simulink model "FeedbackLin"  (R2016a)
settings: Solver=ode45  StartTime=0.0  StopTime=2*Tpasso  FixedStep=1e-4  RelTol=1e-5
values from neighbouring files (symbols this model uses):
  Bm = 1e-4    (= 0.0001)    [runTests.m]
  cm = [c1; c2; c3; c4; c5]    [runTests.m]
  Cphi = 1    [runTests.m]
  cr = [c1; c2; c3; c4; c5]    [runTests.m]
  dQ0 = [dQ10; dQ20; dQ30; dQ40; dQ50]    [runNoErrorNoNoiseNoIncNoFext.m]    (also in runTests.m = zeros(5,1))
  gait = 1    [runTests.m]
  gm = g    (= 9.81)    [runTests.m]
  gr = g    (= 9.81)    [runTests.m]
  Im = [I1; I2; I3; I4; I5]    [runTests.m]
  Ir = [I1; I2; I3; I4; I5]    [runTests.m]
  Jm = 5e-3    (= 0.005)    [runTests.m]
  Kt = 0.1    [runTests.m]
  La = 1e-3    (= 0.001)    [runTests.m]
  LambdaFL = [150; 150; 150; 150]    [runTests.m]
  lm = [l1; l2; l3; l4; l5]    [runTests.m]
  lr = [l1; l2; l3; l4; l5]    [runTests.m]
  mInc = tan(Inc*pi/180)    [runTests.m]
  mm = [m1; m2; m3; m4; m5]    [runTests.m]
  mr = [m1; m2; m3; m4; m5]    [runTests.m]
  pertAmp = 0    [runTests.m]
  pertDur = 0    [runTests.m]
  pertStep = 0    [runTests.m]
  Q0 = [Q10; Q20; Q30; Q40; Q50]    [runNoErrorNoNoiseNoIncNoFext.m]    (also in runTests.m = [pi/2 - pi/10; pi/5; 2*pi-pi/10; pi+pi/10; -pi/4.5])
  Ra = 1    [runTests.m]
  Tpasso = 0.35    [runTests.m]
  TsC = 0.003    [runTests.m]
  TsPID = 1/1000    (= 0.001)    [runTests.m]
  useNoise = false    [runTests.m]
undefined symbols (not defined in the file or in its folder): curStep, Rp1, Rp2
libraries: simulink x8, commrandsrc3 x2
(part 2 of 3)

== matlab function FeedbackLin/calcU ==
  data: Ut output; dQ input; Q input; Yd input; dYd input; ddYd input; Cphi parameter; mm parameter; cm parameter; lm parameter; Im parameter; gm parameter; LambdaFL parameter; Y_bar output
function [Ut, Y_bar] = calcControl(dQ, Q, Yd, dYd, ddYd, Cphi, mm, cm, lm, Im, gm, LambdaFL)
    Mest = zeros(5,5);
    Cest = zeros(5,5);
    Gest = zeros(5,1);
    
    %Control matrices
    diffCq_q    = zeros(4, 5);
    diffLfCq_q  = zeros(4, 5);
    diffLfCq_dq = zeros(4, 5);
    
    %Matrix that appliest 0 torque to joint 1 and the corresponding torque
    %to all other joints.
    Bcontrol = [[0, 0, 0, 0]; ...
                [1, 0, 0, 0]; ...
                [0, 1, 0, 0]; ...
                [0, 0, 1, 0]; ...
                [0, 0, 0, 1]];    
    
    
    %Model Parameters 
    m1 = mm(1);
    m2 = mm(2);
    m3 = mm(3);
    m4 = mm(4);
    m5 = mm(5);

    c1 = cm(1);
    c2 = cm(2);
    c3 = cm(3);
    c4 = cm(4);
    c5 = cm(5);

    l1 = lm(1);
    l2 = lm(2);
    l3 = lm(3);
    l4 = lm(4);
    l5 = lm(5);

    g = gm;

    I1 = Im(1);
    I2 = Im(2);
    I3 = Im(3);
    I4 = Im(4);
    I5 = Im(5);
    
    %Current positions
    q1 = Q(1);
    q2 = Q(2);
    q3 = Q(3);
    q4 = Q(4);
    q5 = Q(5);
    
    dq1 = dQ(1);
    dq2 = dQ(2);
    dq3 = dQ(3);
    dq4 = dQ(4);
    dq5 = dQ(5);
    
    Mest(1, 1) = I1 + I2 + I3 + I4 + I5 + c1^2*m1 + c2^2*m2 + c3^2*m3 + c4^2*m4 + c5^2*m5 + l1^2*m1 + l1^2*m2 + l1^2*m3 + l2^2*m2 + l1^2*m4 + l2^2*m3 + l1^2*m5 + l2^2*m4 + l2^2*m5 + l4^2*m5 - 2*c1*l1*m1 - 2*c2*l2*m2 + 2*c5*l1*m5*cos(q2 + q3 + q4 + q5) + 2*c3*l1*m3*cos(q2 + q3) + 2*c4*l2*m4*cos(q3 + q4) + 2*l2*l4*m5*cos(q3 + q4) - 2*c2*l1*m2*cos(q2) + 2*c3*l2*m3*cos(q3) + 2*c5*l4*m5*cos(q5) + 2*l1*l2*m2*cos(q2) + 2*l1*l2*m3*cos(q2) + 2*l1*l2*m4*cos(q2) + 2*l1*l2*m5*cos(q2) + 2*c4*l1*m4*cos(q2 + q3 + q4) + 2*c5*l2*m5*cos(q3 + q4 + q5) + 2*l1*l4*m5*cos(q2 + q3 + q4);
    Mest(2, 1) = I2 + I3 + I4 + I5 + c2^2*m2 + c3^2*m3 + c4^2*m4 + c5^2*m5 + l2^2*m2 + l2^2*m3 + l2^2*m4 + l2^2*m5 + l4^2*m5 - 2*c2*l2*m2 + c5*l1*m5*cos(q2 + q3 + q4 + q5) + c3*l1*m3*cos(q2 + q3) + 2*c4*l2*m4*cos(q3 + q4) + 2*l2*l4*m5*cos(q3 + q4) - c2*l1*m2*cos(q2) + 2*c3*l2*m3*cos(q3) + 2*c5*l4*m5*cos(q5) + l1*l2*m2*cos(q2) + l1*l2*m3*cos(q2) + l1*l2*m4*cos(q2) + l1*l2*m5*cos(q2) + c4*l1*m4*cos(q2 + q3 + q4) + 2*c5*l2*m5*cos(q3 + q4 + q5) + l1*l4*m5*cos(q2 + q3 + q4);
    Mest(3, 1) = I3 + I4 + I5 + c3^2*m3 + c4^2*m4 + c5^2*m5 + l4^2*m5 + c5*l1*m5*cos(q2 + q3 + q4 + q5) + c3*l1*m3*cos(q2 + q3) + c4*l2*m4*cos(q3 + q4) + l2*l4*m5*cos(q3 + q4) + c3*l2*m3*cos(q3) + 2*c5*l4*m5*cos(q5) + c4*l1*m4*cos(q2 + q3 + q4) + c5*l2*m5*cos(q3 + q4 + q5) + l1*l4*m5*cos(q2 + q3 + q4);
    Mest(4, 1) = I4 + I5 + c4^2*m4 + c5^2*m5 + l4^2*m5 + c5*l1*m5*cos(q2 + q3 + q4 + q5) + c4*l2*m4*cos(q3 + q4) + l2*l4*m5*cos(q3 + q4) + 2*c5*l4*m5*cos(q5) + c4*l1*m4*cos(q2 + q3 + q4) + c5*l2*m5*cos(q3 + q4 + q5) + l1*l4*m5*cos(q2 + q3 + q4);
    Mest(5, 1) = I5 + c5^2*m5 + c5*l1*m5*cos(q2 + q3 + q4 + q5) + c5*l4*m5*cos(q5) + c5*l2*m5*cos(q3 + q4 + q5);
    Mest(1, 2) = I2 + I3 + I4 + I5 + c2^2*m2 + c3^2*m3 + c4^2*m4 + c5^2*m5 + l2^2*m2 + l2^2*m3 + l2^2*m4 + l2^2*m5 + l4^2*m5 - 2*c2*l2*m2 + c5*l1*m5*cos(q2 + q3 + q4 + q5) + c3*l1*m3*cos(q2 + q3) + 2*c4*l2*m4*cos(q3 + q4) + 2*l2*l4*m5*cos(q3 + q4) - c2*l1*m2*cos(q2) + 2*c3*l2*m3*cos(q3) + 2*c5*l4*m5*cos(q5) + l1*l2*m2*cos(q2) + l1*l2*m3*cos(q2) + l1*l2*m4*cos(q2) + l1*l2*m5*cos(q2) + c4*l1*m4*cos(q2 + q3 + q4) + 2*c5*l2*m5*cos(q3 + q4 + q5) + l1*l4*m5*cos(q2 + q3 + q4);
    Mest(2, 2) = I2 + I3 + I4 + I5 + c2^2*m2 + c3^2*m3 + c4^2*m4 + c5^2*m5 + l2^2*m2 + l2^2*m3 + l2^2*m4 + l2^2*m5 + l4^2*m5 - 2*c2*l2*m2 + 2*c4*l2*m4*cos(q3 + q4) + 2*l2*l4*m5*cos(q3 + q4) + 2*c3*l2*m3*cos(q3) + 2*c5*l4*m5*cos(q5) + 2*c5*l2*m5*cos(q3 + q4 + q5);
    Mest(3, 2) = I3 + I4 + I5 + c3^2*m3 + c4^2*m4 + c5^2*m5 + l4^2*m5 + c4*l2*m4*cos(q3 + q4) + l2*l4*m5*cos(q3 + q4) + c3*l2*m3*cos(q3) + 2*c5*l4*m5*cos(q5) + c5*l2*m5*cos(q3 + q4 + q5);
    Mest(4, 2) = I4 + I5 + c4^2*m4 + c5^2*m5 + l4^2*m5 + c4*l2*m4*cos(q3 + q4) + l2*l4*m5*cos(q3 + q4) + 2*c5*l4*m5*cos(q5) + c5*l2*m5*cos(q3 + q4 + q5);
    Mest(5, 2) = I5 + c5^2*m5 + c5*l4*m5*cos(q5) + c5*l2*m5*cos(q3 + q4 + q5);
    Mest(1, 3) = I3 + I4 + I5 + c3^2*m3 + c4^2*m4 + c5^2*m5 + l4^2*m5 + c5*l1*m5*cos(q2 + q3 + q4 + q5) + c3*l1*m3*cos(q2 + q3) + c4*l2*m4*cos(q3 + q4) + l2*l4*m5*cos(q3 + q4) + c3*l2*m3*cos(q3) + 2*c5*l4*m5*cos(q5) + c4*l1*m4*cos(q2 + q3 + q4) + c5*l2*m5*cos(q3 + q4 + q5) + l1*l4*m5*cos(q2 + q3 + q4);
    Mest(2, 3) = I3 + I4 + I5 + c3^2*m3 + c4^2*m4 + c5^2*m5 + l4^2*m5 + c4*l2*m4*cos(q3 + q4) + l2*l4*m5*cos(q3 + q4) + c3*l2*m3*cos(q3) + 2*c5*l4*m5*cos(q5) + c5*l2*m5*cos(q3 + q4 + q5);
    Mest(3, 3) = I3 + I4 + I5 + c3^2*m3 + c4^2*m4 + c5^2*m5 + l4^2*m5 + 2*c5*l4*m5*cos(q5);
    Mest(4, 3) = I4 + I5 + c4^2*m4 + c5^2*m5 + l4^2*m5 + 2*c5*l4*m5*cos(q5);
    Mest(5, 3) = I5 + c5^2*m5 + c5*l4*m5*cos(q5);
    Mest(1, 4) = I4 + I5 + c4^2*m4 + c5^2*m5 + l4^2*m5 + c5*l1*m5*cos(q2 + q3 + q4 + q5) + c4*l2*m4*cos(q3 + q4) + l2*l4*m5*cos(q3 + q4) + 2*c5*l4*m5*cos(q5) + c4*l1*m4*cos(q2 + q3 + q4) + c5*l2*m5*cos(q3 + q4 + q5) + l1*l4*m5*cos(q2 + q3 + q4);
    Mest(2, 4) = I4 + I5 + c4^2*m4 + c5^2*m5 + l4^2*m5 + c4*l2*m4*cos(q3 + q4) + l2*l4*m5*cos(q3 + q4) + 2*c5*l4*m5*cos(q5) + c5*l2*m5*cos(q3 + q4 + q5);
    Mest(3, 4) = I4 + I5 + c4^2*m4 + c5^2*m5 + l4^2*m5 + 2*c5*l4*m5*cos(q5);
    Mest(4, 4) = I4 + I5 + c4^2*m4 + c5^2*m5 + l4^2*m5 + 2*c5*l4*m5*cos(q5);
    Mest(5, 4) = I5 + c5^2*m5 + c5*l4*m5*cos(q5);
    Mest(1, 5) = I5 + c5^2*m5 + c5*l1*m5*cos(q2 + q3 + q4 + q5) + c5*l4*m5*cos(q5) + c5*l2*m5*cos(q3 + q4 + q5);
    Mest(2, 5) = I5 + c5^2*m5 + c5*l4*m5*cos(q5) + c5*l2*m5*cos(q3 + q4 + q5);
    Mest(3, 5) = I5 + c5^2*m5 + c5*l4*m5*cos(q5);
    Mest(4, 5) = I5 + c5^2*m5 + c5*l4*m5*cos(q5);
    Mest(5, 5) = I5 + c5^2*m5;
  
    Gest(1, 1) = g*(m3*(l2*cos(q1 + q2) + l1*cos(q1) + c3*cos(q1 + q2 + q3)) + m5*(l4*cos(q1 + q2 + q3 + q4) + l2*cos(q1 + q2) + l1*cos(q1) + c5*cos(q1 + q2 + q3 + q4 + q5)) - m2*(cos(q1 + q2)*(c2 - l2) - l1*cos(q1)) + m4*(c4*cos(q1 + q2 + q3 + q4) + l2*cos(q1 + q2) + l1*cos(q1)) - m1*cos(q1)*(c1 - l1));
    Gest(2, 1) = g*(m3*(l2*cos(q1 + q2) + c3*cos(q1 + q2 + q3)) + m5*(l4*cos(q1 + q2 + q3 + q4) + l2*cos(q1 + q2) + c5*cos(q1 + q2 + q3 + q4 + q5)) + m4*(c4*cos(q1 + q2 + q3 + q4) + l2*cos(q1 + q2)) - m2*cos(q1 + q2)*(c2 - l2));
    Gest(3, 1) = g*(m5*(l4*cos(q1 + q2 + q3 + q4) + c5*cos(q1 + q2 + q3 + q4 + q5)) + c3*m3*cos(q1 + q2 + q3) + c4*m4*cos(q1 + q2 + q3 + q4));
    Gest(4, 1) = g*(m5*(l4*cos(q1 + q2 + q3 + q4) + c5*cos(q1 + q2 + q3 + q4 + q5)) + c4*m4*cos(q1 + q2 + q3 + q4));
    Gest(5, 1) = c5*g*m5*cos(q1 + q2 + q3 + q4 + q5);
    
    Cest(1, 1) = c2*dq2*l1*m2*sin(q2) - c4*dq3*l1*m4*sin(q2 + q3 + q4) - c4*dq4*l1*m4*sin(q2 + q3 + q4) - c5*dq3*l2*m5*sin(q3 + q4 + q5) - c5*dq4*l2*m5*sin(q3 + q4 + q5) - c5*dq5*l2*m5*sin(q3 + q4 + q5) - dq2*l1*l4*m5*sin(q2 + q3 + q4) - dq3*l1*l4*m5*sin(q2 + q3 + q4) - dq4*l1*l4*m5*sin(q2 + q3 + q4) - c5*dq2*l1*m5*sin(q2 + q3 + q4 + q5) - c5*dq3*l1*m5*sin(q2 + q3 + q4 + q5) - c5*dq4*l1*m5*sin(q2 + q3 + q4 + q5) - c5*dq5*l1*m5*sin(q2 + q3 + q4 + q5) - c3*dq2*l1*m3*sin(q2 + q3) - c3*dq3*l1*m3*sin(q2 + q3) - c4*dq3*l2*m4*sin(q3 + q4) - c4*dq4*l2*m4*sin(q3 + q4) - dq3*l2*l4*m5*sin(q3 + q4) - dq4*l2*l4*m5*sin(q3 + q4) - c4*dq2*l1*m4*sin(q2 + q3 + q4) - c3*dq3*l2*m3*sin(q3) - c5*dq5*l4*m5*sin(q5) - dq2*l1*l2*m2*sin(q2) - dq2*l1*l2*m3*sin(q2) - dq2*l1*l2*m4*sin(q2) - dq2*l1*l2*m5*sin(q2);
    Cest(2, 1) = c4*dq1*l1*m4*sin(q2 + q3 + q4) - c5*dq3*l2*m5*sin(q3 + q4 + q5) - c5*dq4*l2*m5*sin(q3 + q4 + q5) - c5*dq5*l2*m5*sin(q3 + q4 + q5) + dq1*l1*l4*m5*sin(q2 + q3 + q4) + c5*dq1*l1*m5*sin(q2 + q3 + q4 + q5) + c3*dq1*l1*m3*sin(q2 + q3) - c4*dq3*l2*m4*sin(q3 + q4) - c4*dq4*l2*m4*sin(q3 + q4) - dq3*l2*l4*m5*sin(q3 + q4) - dq4*l2*l4*m5*sin(q3 + q4) - c2*dq1*l1*m2*sin(q2) - c3*dq3*l2*m3*sin(q3) - c5*dq5*l4*m5*sin(q5) + dq1*l1*l2*m2*sin(q2) + dq1*l1*l2*m3*sin(q2) + dq1*l1*l2*m4*sin(q2) + dq1*l1*l2*m5*sin(q2);
    Cest(3, 1) = c4*dq1*l1*m4*sin(q2 + q3 + q4) + c5*dq1*l2*m5*sin(q3 + q4 + q5) + c5*dq2*l2*m5*sin(q3 + q4 + q5) + dq1*l1*l4*m5*sin(q2 + q3 + q4) + c5*dq1*l1*m5*sin(q2 + q3 + q4 + q5) + c3*dq1*l1*m3*sin(q2 + q3) + c4*dq1*l2*m4*sin(q3 + q4) + c4*dq2*l2*m4*sin(q3 + q4) + dq1*l2*l4*m5*sin(q3 + q4) + dq2*l2*l4*m5*sin(q3 + q4) + c3*dq1*l2*m3*sin(q3) + c3*dq2*l2*m3*sin(q3) - c5*dq5*l4*m5*sin(q5);
    Cest(4, 1) = c4*dq1*l1*m4*sin(q2 + q3 + q4) + c5*dq1*l2*m5*sin(q3 + q4 + q5) + c5*dq2*l2*m5*sin(q3 + q4 + q5) + dq1*l1*l4*m5*sin(q2 + q3 + q4) + c5*dq1*l1*m5*sin(q2 + q3 + q4 + q5) + c4*dq1*l2*m4*sin(q3 + q4) + c4*dq2*l2*m4*sin(q3 + q4) + dq1*l2*l4*m5*sin(q3 + q4) + dq2*l2*l4*m5*sin(q3 + q4) - c5*dq5*l4*m5*sin(q5);
    Cest(5, 1) = c5*m5*(dq1*l4*sin(q5) + dq2*l4*sin(q5) + dq3*l4*sin(q5) + dq4*l4*sin(q5) + dq1*l2*sin(q3 + q4 + q5) + dq2*l2*sin(q3 + q4 + q5) + dq1*l1*sin(q2 + q3 + q4 + q5));
    Cest(1, 2) = c2*dq1*l1*m2*sin(q2) - c4*dq2*l1*m4*sin(q2 + q3 + q4) - c4*dq3*l1*m4*sin(q2 + q3 + q4) - c4*dq4*l1*m4*sin(q2 + q3 + q4) - c5*dq3*l2*m5*sin(q3 + q4 + q5) - c5*dq4*l2*m5*sin(q3 + q4 + q5) - c5*dq5*l2*m5*sin(q3 + q4 + q5) - dq1*l1*l4*m5*sin(q2 + q3 + q4) - dq2*l1*l4*m5*sin(q2 + q3 + q4) - dq3*l1*l4*m5*sin(q2 + q3 + q4) - dq4*l1*l4*m5*sin(q2 + q3 + q4) - c5*dq1*l1*m5*sin(q2 + q3 + q4 + q5) - c5*dq2*l1*m5*sin(q2 + q3 + q4 + q5) - c5*dq3*l1*m5*sin(q2 + q3 + q4 + q5) - c5*dq4*l1*m5*sin(q2 + q3 + q4 + q5) - c5*dq5*l1*m5*sin(q2 + q3 + q4 + q5) - c3*dq1*l1*m3*sin(q2 + q3) - c3*dq2*l1*m3*sin(q2 + q3) - c3*dq3*l1*m3*sin(q2 + q3) - c4*dq3*l2*m4*sin(q3 + q4) - c4*dq4*l2*m4*sin(q3 + q4) - dq3*l2*l4*m5*sin(q3 + q4) - dq4*l2*l4*m5*sin(q3 + q4) - c4*dq1*l1*m4*sin(q2 + q3 + q4) + c2*dq2*l1*m2*sin(q2) - c3*dq3*l2*m3*sin(q3) - c5*dq5*l4*m5*sin(q5) - dq1*l1*l2*m2*sin(q2) - dq1*l1*l2*m3*sin(q2) - dq2*l1*l2*m2*sin(q2) - dq1*l1*l2*m4*sin(q2) - dq2*l1*l2*m3*sin(q2) - dq1*l1*l2*m5*sin(q2) - dq2*l1*l2*m4*sin(q2) - dq2*l1*l2*m5*sin(q2);
    Cest(2, 2) = - dq4*l2*(c5*m5*sin(q3 + q4 + q5) + c4*m4*sin(q3 + q4) + l4*m5*sin(q3 + q4)) - dq3*l2*(c3*m3*sin(q3) + c5*m5*sin(q3 + q4 + q5) + c4*m4*sin(q3 + q4) + l4*m5*sin(q3 + q4)) - c5*dq5*m5*(l4*sin(q5) + l2*sin(q3 + q4 + q5));
    Cest(3, 2) = c5*dq1*l2*m5*sin(q3 + q4 + q5) + c5*dq2*l2*m5*sin(q3 + q4 + q5) + c4*dq1*l2*m4*sin(q3 + q4) + c4*dq2*l2*m4*sin(q3 + q4) + dq1*l2*l4*m5*sin(q3 + q4) + dq2*l2*l4*m5*sin(q3 + q4) + c3*dq1*l2*m3*sin(q3) + c3*dq2*l2*m3*sin(q3) - c5*dq5*l4*m5*sin(q5);
    Cest(4, 2) = c5*dq1*l2*m5*sin(q3 + q4 + q5) + c5*dq2*l2*m5*sin(q3 + q4 + q5) + c4*dq1*l2*m4*sin(q3 + q4) + c4*dq2*l2*m4*sin(q3 + q4) + dq1*l2*l4*m5*sin(q3 + q4) + dq2*l2*l4*m5*sin(q3 + q4) - c5*dq5*l4*m5*sin(q5);
    Cest(5, 2) = c5*m5*(dq1*l4*sin(q5) + dq2*l4*sin(q5) + dq3*l4*sin(q5) + dq4*l4*sin(q5) + dq1*l2*sin(q3 + q4 + q5) + dq2*l2*sin(q3 + q4 + q5));
    Cest(1, 3) = - c4*dq1*l1*m4*sin(q2 + q3 + q4) - c4*dq2*l1*m4*sin(q2 + q3 + q4) - c4*dq3*l1*m4*sin(q2 + q3 + q4) - c4*dq4*l1*m4*sin(q2 + q3 + q4) - c5*dq1*l2*m5*sin(q3 + q4 + q5) - c5*dq2*l2*m5*sin(q3 + q4 + q5) - c5*dq3*l2*m5*sin(q3 + q4 + q5) - c5*dq4*l2*m5*sin(q3 + q4 + q5) - c5*dq5*l2*m5*sin(q3 + q4 + q5) - dq1*l1*l4*m5*sin(q2 + q3 + q4) - dq2*l1*l4*m5*sin(q2 + q3 + q4) - dq3*l1*l4*m5*sin(q2 + q3 + q4) - dq4*l1*l4*m5*sin(q2 + q3 + q4) - c5*dq1*l1*m5*sin(q2 + q3 + q4 + q5) - c5*dq2*l1*m5*sin(q2 + q3 + q4 + q5) - c5*dq3*l1*m5*sin(q2 + q3 + q4 + q5) - c5*dq4*l1*m5*sin(q2 + q3 + q4 + q5) - c5*dq5*l1*m5*sin(q2 + q3 + q4 + q5) - c3*dq1*l1*m3*sin(q2 + q3) - c3*dq2*l1*m3*sin(q2 + q3) - c3*dq3*l1*m3*sin(q2 + q3) - c4*dq1*l2*m4*sin(q3 + q4) - c4*dq2*l2*m4*sin(q3 + q4) - c4*dq3*l2*m4*sin(q3 + q4) - c4*dq4*l2*m4*sin(q3 + q4) - dq1*l2*l4*m5*sin(q3 + q4) - dq2*l2*l4*m5*sin(q3 + q4) - dq3*l2*l4*m5*sin(q3 + q4) - dq4*l2*l4*m5*sin(q3 + q4) - c3*dq1*l2*m3*sin(q3) - c3*dq2*l2*m3*sin(q3) - c3*dq3*l2*m3*sin(q3) - c5*dq5*l4*m5*sin(q5);
    Cest(2, 3) = - c5*dq1*l2*m5*sin(q3 + q4 + q5) - c5*dq2*l2*m5*sin(q3 + q4 + q5) - c5*dq3*l2*m5*sin(q3 + q4 + q5) - c5*dq4*l2*m5*sin(q3 + q4 + q5) - c5*dq5*l2*m5*sin(q3 + q4 + q5) - c4*dq1*l2*m4*sin(q3 + q4) - c4*dq2*l2*m4*sin(q3 + q4) - c4*dq3*l2*m4*sin(q3 + q4) - c4*dq4*l2*m4*sin(q3 + q4) - dq1*l2*l4*m5*sin(q3 + q4) - dq2*l2*l4*m5*sin(q3 + q4) - dq3*l2*l4*m5*sin(q3 + q4) - dq4*l2*l4*m5*sin(q3 + q4) - c3*dq1*l2*m3*sin(q3) - c3*dq2*l2*m3*sin(q3) - c3*dq3*l2*m3*sin(q3) - c5*dq5*l4*m5*sin(q5);
    Cest(3, 3) = -c5*dq5*l4*m5*sin(q5);
    Cest(4, 3) = -c5*dq5*l4*m5*sin(q5);
    Cest(5, 3) = c5*l4*m5*sin(q5)*(dq1 + dq2 + dq3 + dq4);
    Cest(1, 4) = - c4*dq1*l1*m4*sin(q2 + q3 + q4) - c4*dq2*l1*m4*sin(q2 + q3 + q4) - c4*dq3*l1*m4*sin(q2 + q3 + q4) - c4*dq4*l1*m4*sin(q2 + q3 + q4) - c5*dq1*l2*m5*sin(q3 + q4 + q5) - c5*dq2*l2*m5*sin(q3 + q4 + q5) - c5*dq3*l2*m5*sin(q3 + q4 + q5) - c5*dq4*l2*m5*sin(q3 + q4 + q5) - c5*dq5*l2*m5*sin(q3 + q4 + q5) - dq1*l1*l4*m5*sin(q2 + q3 + q4) - dq2*l1*l4*m5*sin(q2 + q3 + q4) - dq3*l1*l4*m5*sin(q2 + q3 + q4) - dq4*l1*l4*m5*sin(q2 + q3 + q4) - c5*dq1*l1*m5*sin(q2 + q3 + q4 + q5) - c5*dq2*l1*m5*sin(q2 + q3 + q4 + q5) - c5*dq3*l1*m5*sin(q2 + q3 + q4 + q5) - c5*dq4*l1*m5*sin(q2 + q3 + q4 + q5) - c5*dq5*l1*m5*sin(q2 + q3 + q4 + q5) - c4*dq1*l2*m4*sin(q3 + q4) - c4*dq2*l2*m4*sin(q3 + q4) - c4*dq3*l2*m4*sin(q3 + q4) - c4*dq4*l2*m4*sin(q3 + q4) - dq1*l2*l4*m5*sin(q3 + q4) - dq2*l2*l4*m5*sin(q3 + q4) - dq3*l2*l4*m5*sin(q3 + q4) - dq4*l2*l4*m5*sin(q3 + q4) - c5*dq5*l4*m5*sin(q5);
    Cest(2, 4) = - c5*dq1*l2*m5*sin(q3 + q4 + q5) - c5*dq2*l2*m5*sin(q3 + q4 + q5) - c5*dq3*l2*m5*sin(q3 + q4 + q5) - c5*dq4*l2*m5*sin(q3 + q4 + q5) - c5*dq5*l2*m5*sin(q3 + q4 + q5) - c4*dq1*l2*m4*sin(q3 + q4) - c4*dq2*l2*m4*sin(q3 + q4) - c4*dq3*l2*m4*sin(q3 + q4) - c4*dq4*l2*m4*sin(q3 + q4) - dq1*l2*l4*m5*sin(q3 + q4) - dq2*l2*l4*m5*sin(q3 + q4) - dq3*l2*l4*m5*sin(q3 + q4) - dq4*l2*l4*m5*sin(q3 + q4) - c5*dq5*l4*m5*sin(q5);
    Cest(3, 4) = -c5*dq5*l4*m5*sin(q5);
    Cest(4, 4) = -c5*dq5*l4*m5*sin(q5);
    Cest(5, 4) = c5*l4*m5*sin(q5)*(dq1 + dq2 + dq3 + dq4);
    Cest(1, 5) = -c5*m5*(l1*sin(q2 + q3 + q4 + q5) + l4*sin(q5) + l2*sin(q3 + q4 + q5))*(dq1 + dq2 + dq3 + dq4 + dq5);
    Cest(2, 5) = -c5*m5*(l4*sin(q5) + l2*sin(q3 + q4 + q5))*(dq1 + dq2 + dq3 + dq4 + dq5);
    Cest(3, 5) = -c5*l4*m5*sin(q5)*(dq1 + dq2 + dq3 + dq4 + dq5);
    Cest(4, 5) = -c5*l4*m5*sin(q5)*(dq1 + dq2 + dq3 + dq4 + dq5);
    Cest(5, 5) = 0;
    
    %Control Matrices
    Ffric = Cphi*[0; dq2; dq3; dq4; dq5];
    
    f1 = [dq1; dq2; dq3; dq4; dq5];
    f2 = -Mest\(Cest*[dq1; dq2; dq3; dq4; dq5] + Gest + Ffric);
    
    g2 = Mest\Bcontrol;
    
    %Lie Derivatives
    diffCq_q(1, 1) = -1;
    diffCq_q(2, 1) = l4*cos(q1 + q2 + q3 + q4) + l2*cos(q1 + q2) + l1*cos(q1) + l5*cos(q1 + q2 + q3 + q4 + q5);
    diffCq_q(3, 1) = (m3*(l2*cos(q1 + q2) + l1*cos(q1) + c3*cos(q1 + q2 + q3)) + m5*(l4*cos(q1 + q2 + q3 + q4) + l2*cos(q1 + q2) + l1*cos(q1) + c5*cos(q1 + q2 + q3 + q4 + q5)) - m2*(cos(q1 + q2)*(c2 - l2) - l1*cos(q1)) + m4*(c4*cos(q1 + q2 + q3 + q4) + l2*cos(q1 + q2) + l1*cos(q1)) - m1*cos(q1)*(c1 - l1))/(m1 + m2 + m3 + m4 + m5);
    diffCq_q(4, 1) = - l4*sin(q1 + q2 + q3 + q4) - l2*sin(q1 + q2) - l1*sin(q1) - l5*sin(q1 + q2 + q3 + q4 + q5);
    diffCq_q(1, 2) = -1;
    diffCq_q(2, 2) = l4*cos(q1 + q2 + q3 + q4) + l2*cos(q1 + q2) + l5*cos(q1 + q2 + q3 + q4 + q5);
    diffCq_q(3, 2) = (m3*(l2*cos(q1 + q2) + c3*cos(q1 + q2 + q3)) + m5*(l4*cos(q1 + q2 + q3 + q4) + l2*cos(q1 + q2) + c5*cos(q1 + q2 + q3 + q4 + q5)) + m4*(c4*cos(q1 + q2 + q3 + q4) + l2*cos(q1 + q2)) - m2*cos(q1 + q2)*(c2 - l2))/(m1 + m2 + m3 + m4 + m5);
    diffCq_q(4, 2) = - l4*sin(q1 + q2 + q3 + q4) - l2*sin(q1 + q2) - l5*sin(q1 + q2 + q3 + q4 + q5);
    diffCq_q(1, 3) = -1;
    diffCq_q(2, 3) = l4*cos(q1 + q2 + q3 + q4) + l5*cos(q1 + q2 + q3 + q4 + q5);
    diffCq_q(3, 3) = (m5*(l4*cos(q1 + q2 + q3 + q4) + c5*cos(q1 + q2 + q3 + q4 + q5)) + c3*m3*cos(q1 + q2 + q3) + c4*m4*cos(q1 + q2 + q3 + q4))/(m1 + m2 + m3 + m4 + m5);
    diffCq_q(4, 3) = - l4*sin(q1 + q2 + q3 + q4) - l5*sin(q1 + q2 + q3 + q4 + q5);
    diffCq_q(1, 4) = 0;
    diffCq_q(2, 4) = l4*cos(q1 + q2 + q3 + q4) + l5*cos(q1 + q2 + q3 + q4 + q5);
    diffCq_q(3, 4) = (m5*(l4*cos(q1 + q2 + q3 + q4) + c5*cos(q1 + q2 + q3 + q4 + q5)) + c4*m4*cos(q1 + q2 + q3 + q4))/(m1 + m2 + m3 + m4 + m5);
    diffCq_q(4, 4) = - l4*sin(q1 + q2 + q3 + q4) - l5*sin(q1 + q2 + q3 + q4 + q5);
    diffCq_q(1, 5) = 0;
    diffCq_q(2, 5) = l5*cos(q1 + q2 + q3 + q4 + q5);
    diffCq_q(3, 5) = (c5*m5*cos(q1 + q2 + q3 + q4 + q5))/(m1 + m2 + m3 + m4 + m5);
    diffCq_q(4, 5) = -l5*sin(q1 + q2 + q3 + q4 + q5);
    
    diffLfCq_q(1, 1) = 0;
    diffLfCq_q(2, 1) = - dq3*(l4*sin(q1 + q2 + q3 + q4) + l5*sin(q1 + q2 + q3 + q4 + q5)) - dq4*(l4*sin(q1 + q2 + q3 + q4) + l5*sin(q1 + q2 + q3 + q4 + q5)) - dq1*(l4*sin(q1 + q2 + q3 + q4) + l2*sin(q1 + q2) + l1*sin(q1) + l5*sin(q1 + q2 + q3 + q4 + q5)) - dq2*(l4*sin(q1 + q2 + q3 + q4) + l2*sin(q1 + q2) + l5*sin(q1 + q2 + q3 + q4 + q5)) - dq5*l5*sin(q1 + q2 + q3 + q4 + q5);
    diffLfCq_q(3, 1) = - (dq4*(m5*(l4*sin(q1 + q2 + q3 + q4) + c5*sin(q1 + q2 + q3 + q4 + q5)) + c4*m4*sin(q1 + q2 + q3 + q4)))/(m1 + m2 + m3 + m4 + m5) - (dq1*(m3*(l2*sin(q1 + q2) + l1*sin(q1) + c3*sin(q1 + q2 + q3)) - m2*(sin(q1 + q2)*(c2 - l2) - l1*sin(q1)) + m5*(l4*sin(q1 + q2 + q3 + q4) + l2*sin(q1 + q2) + l1*sin(q1) + c5*sin(q1 + q2 + q3 + q4 + q5)) + m4*(c4*sin(q1 + q2 + q3 + q4) + l2*sin(q1 + q2) + l1*sin(q1)) - m1*sin(q1)*(c1 - l1)))/(m1 + m2 + m3 + m4 + m5) - (dq3*(m5*(l4*sin(q1 + q2 + q3 + q4) + c5*sin(q1 + q2 + q3 + q4 + q5)) + c3*m3*sin(q1 + q2 + q3) + c4*m4*sin(q1 + q2 + q3 + q4)))/(m1 + m2 + m3 + m4 + m5) - (dq2*(m4*(c4*sin(q1 + q2 + q3 + q4) + l2*sin(q1 + q2)) + m3*(l2*sin(q1 + q2) + c3*sin(q1 + q2 + q3)) + m5*(l4*sin(q1 + q2 + q3 + q4) + l2*sin(q1 + q2) + c5*sin(q1 + q2 + q3 + q4 + q5)) - m2*sin(q1 + q2)*(c2 - l2)))/(m1 + m2 + m3 + m4 + m5) - (c5*dq5*m5*sin(q1 + q2 + q3 + q4 + q5))/(m1 + m2 + m3 + m4 + m5);
    diffLfCq_q(4, 1) = - dq3*(l4*cos(q1 + q2 + q3 + q4) + l5*cos(q1 + q2 + q3 + q4 + q5)) - dq4*(l4*cos(q1 + q2 + q3 + q4) + l5*cos(q1 + q2 + q3 + q4 + q5)) - dq1*(l4*cos(q1 + q2 + q3 + q4) + l2*cos(q1 + q2) + l1*cos(q1) + l5*cos(q1 + q2 + q3 + q4 + q5)) - dq2*(l4*cos(q1 + q2 + q3 + q4) + l2*cos(q1 + q2) + l5*cos(q1 + q2 + q3 + q4 + q5)) - dq5*l5*cos(q1 + q2 + q3 + q4 + q5);
    diffLfCq_q(1, 2) = 0;
    diffLfCq_q(2, 2) = - dq3*(l4*sin(q1 + q2 + q3 + q4) + l5*sin(q1 + q2 + q3 + q4 + q5)) - dq4*(l4*sin(q1 + q2 + q3 + q4) + l5*sin(q1 + q2 + q3 + q4 + q5)) - dq1*(l4*sin(q1 + q2 + q3 + q4) + l2*sin(q1 + q2) + l5*sin(q1 + q2 + q3 + q4 + q5)) - dq2*(l4*sin(q1 + q2 + q3 + q4) + l2*sin(q1 + q2) + l5*sin(q1 + q2 + q3 + q4 + q5)) - dq5*l5*sin(q1 + q2 + q3 + q4 + q5);
    diffLfCq_q(3, 2) = - (dq4*(m5*(l4*sin(q1 + q2 + q3 + q4) + c5*sin(q1 + q2 + q3 + q4 + q5)) + c4*m4*sin(q1 + q2 + q3 + q4)))/(m1 + m2 + m3 + m4 + m5) - (dq3*(m5*(l4*sin(q1 + q2 + q3 + q4) + c5*sin(q1 + q2 + q3 + q4 + q5)) + c3*m3*sin(q1 + q2 + q3) + c4*m4*sin(q1 + q2 + q3 + q4)))/(m1 + m2 + m3 + m4 + m5) - (dq1*(m4*(c4*sin(q1 + q2 + q3 + q4) + l2*sin(q1 + q2)) + m3*(l2*sin(q1 + q2) + c3*sin(q1 + q2 + q3)) + m5*(l4*sin(q1 + q2 + q3 + q4) + l2*sin(q1 + q2) + c5*sin(q1 + q2 + q3 + q4 + q5)) - m2*sin(q1 + q2)*(c2 - l2)))/(m1 + m2 + m3 + m4 + m5) - (dq2*(m4*(c4*sin(q1 + q2 + q3 + q4) + l2*sin(q1 + q2)) + m3*(l2*sin(q1 + q2) + c3*sin(q1 + q2 + q3)) + m5*(l4*sin(q1 + q2 + q3 + q4) + l2*sin(q1 + q2) + c5*sin(q1 + q2 + q3 + q4 + q5)) - m2*sin(q1 + q2)*(c2 - l2)))/(m1 + m2 + m3 + m4 + m5) - (c5*dq5*m5*sin(q1 + q2 + q3 + q4 + q5))/(m1 + m2 + m3 + m4 + m5);
    diffLfCq_q(4, 2) = - dq3*(l4*cos(q1 + q2 + q3 + q4) + l5*cos(q1 + q2 + q3 + q4 + q5)) - dq4*(l4*cos(q1 + q2 + q3 + q4) + l5*cos(q1 + q2 + q3 + q4 + q5)) - dq1*(l4*cos(q1 + q2 + q3 + q4) + l2*cos(q1 + q2) + l5*cos(q1 + q2 + q3 + q4 + q5)) - dq2*(l4*cos(q1 + q2 + q3 + q4) + l2*cos(q1 + q2) + l5*cos(q1 + q2 + q3 + q4 + q5)) - dq5*l5*cos(q1 + q2 + q3 + q4 + q5);
    diffLfCq_q(1, 3) = 0;
    diffLfCq_q(2, 3) = - dq1*(l4*sin(q1 + q2 + q3 + q4) + l5*sin(q1 + q2 + q3 + q4 + q5)) - dq2*(l4*sin(q1 + q2 + q3 + q4) + l5*sin(q1 + q2 + q3 + q4 + q5)) - dq3*(l4*sin(q1 + q2 + q3 + q4) + l5*sin(q1 + q2 + q3 + q4 + q5)) - dq4*(l4*sin(q1 + q2 + q3 + q4) + l5*sin(q1 + q2 + q3 + q4 + q5)) - dq5*l5*sin(q1 + q2 + q3 + q4 + q5);
    diffLfCq_q(3, 3) = -(c4*dq1*m4*sin(q1 + q2 + q3 + q4) + c4*dq2*m4*sin(q1 + q2 + q3 + q4) + c4*dq3*m4*sin(q1 + q2 + q3 + q4) + c4*dq4*m4*sin(q1 + q2 + q3 + q4) + dq1*l4*m5*sin(q1 + q2 + q3 + q4) + dq2*l4*m5*sin(q1 + q2 + q3 + q4) + dq3*l4*m5*sin(q1 + q2 + q3 + q4) + dq4*l4*m5*sin(q1 + q2 + q3 + q4) + c5*dq1*m5*sin(q1 + q2 + q3 + q4 + q5) + c5*dq2*m5*sin(q1 + q2 + q3 + q4 + q5) + c5*dq3*m5*sin(q1 + q2 + q3 + q4 + q5) + c5*dq4*m5*sin(q1 + q2 + q3 + q4 + q5) + c5*dq5*m5*sin(q1 + q2 + q3 + q4 + q5) + c3*dq1*m3*sin(q1 + q2 + q3) + c3*dq2*m3*sin(q1 + q2 + q3) + c3*dq3*m3*sin(q1 + q2 + q3))/(m1 + m2 + m3 + m4 + m5);
    diffLfCq_q(4, 3) = - dq1*(l4*cos(q1 + q2 + q3 + q4) + l5*cos(q1 + q2 + q3 + q4 + q5)) - dq2*(l4*cos(q1 + q2 + q3 + q4) + l5*cos(q1 + q2 + q3 + q4 + q5)) - dq3*(l4*cos(q1 + q2 + q3 + q4) + l5*cos(q1 + q2 + q3 + q4 + q5)) - dq4*(l4*cos(q1 + q2 + q3 + q4) + l5*cos(q1 + q2 + q3 + q4 + q5)) - dq5*l5*cos(q1 + q2 + q3 + q4 + q5);
    diffLfCq_q(1, 4) = 0;
    diffLfCq_q(2, 4) = - dq1*(l4*sin(q1 + q2 + q3 + q4) + l5*sin(q1 + q2 + q3 + q4 + q5)) - dq2*(l4*sin(q1 + q2 + q3 + q4) + l5*sin(q1 + q2 + q3 + q4 + q5)) - dq3*(l4*sin(q1 + q2 + q3 + q4) + l5*sin(q1 + q2 + q3 + q4 + q5)) - dq4*(l4*sin(q1 + q2 + q3 + q4) + l5*sin(q1 + q2 + q3 + q4 + q5)) - dq5*l5*sin(q1 + q2 + q3 + q4 + q5);
    diffLfCq_q(3, 4) = -(c4*dq1*m4*sin(q1 + q2 + q3 + q4) + c4*dq2*m4*sin(q1 + q2 + q3 + q4) + c4*dq3*m4*sin(q1 + q2 + q3 + q4) + c4*dq4*m4*sin(q1 + q2 + q3 + q4) + dq1*l4*m5*sin(q1 + q2 + q3 + q4) + dq2*l4*m5*sin(q1 + q2 + q3 + q4) + dq3*l4*m5*sin(q1 + q2 + q3 + q4) + dq4*l4*m5*sin(q1 + q2 + q3 + q4) + c5*dq1*m5*sin(q1 + q2 + q3 + q4 + q5) + c5*dq2*m5*sin(q1 + q2 + q3 + q4 + q5) + c5*dq3*m5*sin(q1 + q2 + q3 + q4 + q5) + c5*dq4*m5*sin(q1 + q2 + q3 + q4 + q5) + c5*dq5*m5*sin(q1 + q2 + q3 + q4 + q5))/(m1 + m2 + m3 + m4 + m5);
    diffLfCq_q(4, 4) = - dq1*(l4*cos(q1 + q2 + q3 + q4) + l5*cos(q1 + q2 + q3 + q4 + q5)) - dq2*(l4*cos(q1 + q2 + q3 + q4) + l5*cos(q1 + q2 + q3 + q4 + q5)) - dq3*(l4*cos(q1 + q2 + q3 + q4) + l5*cos(q1 + q2 + q3 + q4 + q5)) - dq4*(l4*cos(q1 + q2 + q3 + q4) + l5*cos(q1 + q2 + q3 + q4 + q5)) - dq5*l5*cos(q1 + q2 + q3 + q4 + q5);
    diffLfCq_q(1, 5) = 0;
    diffLfCq_q(2, 5) = -l5*sin(q1 + q2 + q3 + q4 + q5)*(dq1 + dq2 + dq3 + dq4 + dq5);
    diffLfCq_q(3, 5) = -(c5*m5*sin(q1 + q2 + q3 + q4 + q5)*(dq1 + dq2 + dq3 + dq4 + dq5))/(m1 + m2 + m3 + m4 + m5);
    diffLfCq_q(4, 5) = -l5*cos(q1 + q2 + q3 + q4 + q5)*(dq1 + dq2 + dq3 + dq4 + dq5);
    
    diffLfCq_dq(1, 1) = -1;
    diffLfCq_dq(2, 1) = l4*cos(q1 + q2 + q3 + q4) + l2*cos(q1 + q2) + l1*cos(q1) + l5*cos(q1 + q2 + q3 + q4 + q5);
    diffLfCq_dq(3, 1) = (m3*(l2*cos(q1 + q2) + l1*cos(q1) + c3*cos(q1 + q2 + q3)) + m5*(l4*cos(q1 + q2 + q3 + q4) + l2*cos(q1 + q2) + l1*cos(q1) + c5*cos(q1 + q2 + q3 + q4 + q5)) - m2*(cos(q1 + q2)*(c2 - l2) - l1*cos(q1)) + m4*(c4*cos(q1 + q2 + q3 + q4) + l2*cos(q1 + q2) + l1*cos(q1)) - m1*cos(q1)*(c1 - l1))/(m1 + m2 + m3 + m4 + m5);
    diffLfCq_dq(4, 1) = - l4*sin(q1 + q2 + q3 + q4) - l2*sin(q1 + q2) - l1*sin(q1) - l5*sin(q1 + q2 + q3 + q4 + q5);
    diffLfCq_dq(1, 2) = -1;
    diffLfCq_dq(2, 2) = l4*cos(q1 + q2 + q3 + q4) + l2*cos(q1 + q2) + l5*cos(q1 + q2 + q3 + q4 + q5);
    diffLfCq_dq(3, 2) = (m3*(l2*cos(q1 + q2) + c3*cos(q1 + q2 + q3)) + m5*(l4*cos(q1 + q2 + q3 + q4) + l2*cos(q1 + q2) + c5*cos(q1 + q2 + q3 + q4 + q5)) + m4*(c4*cos(q1 + q2 + q3 + q4) + l2*cos(q1 + q2)) - m2*cos(q1 + q2)*(c2 - l2))/(m1 + m2 + m3 + m4 + m5);
    diffLfCq_dq(4, 2) = - l4*sin(q1 + q2 + q3 + q4) - l2*sin(q1 + q2) - l5*sin(q1 + q2 + q3 + q4 + q5);
    diffLfCq_dq(1, 3) = -1;
    diffLfCq_dq(2, 3) = l4*cos(q1 + q2 + q3 + q4) + l5*cos(q1 + q2 + q3 + q4 + q5);
    diffLfCq_dq(3, 3) = (m5*(l4*cos(q1 + q2 + q3 + q4) + c5*cos(q1 + q2 + q3 + q4 + q5)) + c3*m3*cos(q1 + q2 + q3) + c4*m4*cos(q1 + q2 + q3 + q4))/(m1 + m2 + m3 + m4 + m5);
    diffLfCq_dq(4, 3) = - l4*sin(q1 + q2 + q3 + q4) - l5*sin(q1 + q2 + q3 + q4 + q5);
    diffLfCq_dq(1, 4) = 0;
    diffLfCq_dq(2, 4) = l4*cos(q1 + q2 + q3 + q4) + l5*cos(q1 + q2 + q3 + q4 + q5);
    diffLfCq_dq(3, 4) = (m5*(l4*cos(q1 + q2 + q3 + q4) + c5*cos(q1 + q2 + q3 + q4 + q5)) + c4*m4*cos(q1 + q2 + q3 + q4))/(m1 + m2 + m3 + m4 + m5);
    diffLfCq_dq(4, 4) = - l4*sin(q1 + q2 + q3 + q4) - l5*sin(q1 + q2 + q3 + q4 + q5);
    diffLfCq_dq(1, 5) = 0;
    diffLfCq_dq(2, 5) = l5*cos(q1 + q2 + q3 + q4 + q5);
    diffLfCq_dq(3, 5) = (c5*m5*cos(q1 + q2 + q3 + q4 + q5))/(m1 + m2 + m3 + m4 + m5);
    diffLfCq_dq(4, 5) = -l5*sin(q1 + q2 + q3 + q4 + q5);
    
    LfCq    = diffCq_q*f1;
    Lf_2_Cq = diffLfCq_q*f1 + diffLfCq_dq*f2;
    LgLfCq  = diffLfCq_dq*g2;
    
    %%% Control Parameters
    %There is no longer 5 terms for the control, since only 4 of the joints
    %are actuated.
    
    %Form of Y (dY is already calculated as LfCq)
    Y_bar = zeros(4, 1);
    
    Y_bar(1) = ((5*pi/2) - q1 - q2 - q3);
    Y_bar(2) = (l1*sin(q1) + l2*sin(q1+q2) + l4*sin(q1+q2+q3+q4) + l5*sin(q1+q2+q3+q4+q5));
    Y_bar(3) = (m3*(l2*sin(q1 + q2) + l1*sin(q1) + c3*sin(q1 + q2 + q3)) - m2*(sin(q1 + q2)*(c2 - l2) - l1*sin(q1)) + m5*(l4*sin(q1 + q2 + q3 + q4) + l2*sin(q1 + q2) + l1*sin(q1) + c5*sin(q1 + q2 + q3 + q4 + q5)) + m4*(c4*sin(q1 + q2 + q3 + q4) + l2*sin(q1 + q2) + l1*sin(q1)) - m1*sin(q1)*(c1 - l1))/(m1 + m2 + m3 + m4 + m5);
    Y_bar(4) = (l1*cos(q1) + l2*cos(q1+q2) + l4*cos(q1+q2+q3+q4) + l5*cos(q1+q2+q3+q4+q5));
    
    %Lambda of the PD
    lambda = diag([LambdaFL(1), LambdaFL(2), LambdaFL(3), LambdaFL(4)]);
    
    %Computation of v
    v = ddYd - 2*lambda*(LfCq - dYd) - lambda*lambda*(Y_bar - Yd);
    
    %Computation of the final control input
    U = LgLfCq\(v - Lf_2_Cq);
    
    %Finally, adds the zero torque virtual control of joint 1. This is done
    %just to use the same architecture as all other simulations;
    Ut = [0;U];
end

== matlab function FeedbackLin/Rabbit ==
  data: U input; Q input; ddQ output; dQ input; fext input; Qext output; momentum output; Cphi parameter; mr parameter; cr parameter; lr parameter; Ir parameter; gr parameter; U output
function [ddQ, Qext, momentum, U] = model(U, Q, dQ, fext, Cphi, mr, cr, lr, Ir, gr)
    M = zeros(5,5);
    C = zeros(5,1);
    G = zeros(5,1);
    Qext = zeros(5,1);
    
    %Model Params
    m1 = mr(1);
    m2 = mr(2);
    m3 = mr(3);
    m4 = mr(4);
    m5 = mr(5);

    c1 = cr(1);
    c2 = cr(2);
    c3 = cr(3);
    c4 = cr(4);
    c5 = cr(5);

    l1 = lr(1);
    l2 = lr(2);
    l3 = lr(3);
    l4 = lr(4);
    l5 = lr(5);

    g = gr;

    I1 = Ir(1);
    I2 = Ir(2);
    I3 = Ir(3);
    I4 = Ir(4);
    I5 = Ir(5);
    
    q1 = Q(1);
    q2 = Q(2);
    q3 = Q(3);
    q4 = Q(4);
    q5 = Q(5);
    
    dq1 = dQ(1);
    dq2 = dQ(2);
    dq3 = dQ(3);
    dq4 = dQ(4);
    dq5 = dQ(5);
    
    F1  = fext(1);
    F2  = fext(2);
    F3  = fext(3);
    F4  = fext(4);
    F5  = fext(5);
    F6  = fext(6);
    F7  = fext(7);
    F8  = fext(8);
    F9  = fext(9);
    F10 = fext(10);
    
    F11 = fext(11);
    F12 = fext(12);
    F13 = fext(13);
    F14 = fext(14);
    F15 = fext(15);
    
    M(1,1) = I1 + I2 + I3 + I4 + I5 + c1^2*m1 + c2^2*m2 + c3^2*m3 + c4^2*m4 + c5^2*m5 + l1^2*m1 + l1^2*m2 + l1^2*m3 + l2^2*m2 + l1^2*m4 + l2^2*m3 + l1^2*m5 + l2^2*m4 + l2^2*m5 + l4^2*m5 - 2*c1*l1*m1 - 2*c2*l2*m2 + 2*c5*l1*m5*cos(q2 + q3 + q4 + q5) + 2*c3*l1*m3*cos(q2 + q3) + 2*c4*l2*m4*cos(q3 + q4) + 2*l2*l4*m5*cos(q3 + q4) - 2*c2*l1*m2*cos(q2) + 2*c3*l2*m3*cos(q3) + 2*c5*l4*m5*cos(q5) + 2*l1*l2*m2*cos(q2) + 2*l1*l2*m3*cos(q2) + 2*l1*l2*m4*cos(q2) + 2*l1*l2*m5*cos(q2) + 2*c4*l1*m4*cos(q2 + q3 + q4) + 2*c5*l2*m5*cos(q3 + q4 + q5) + 2*l1*l4*m5*cos(q2 + q3 + q4);
    M(1,2) = I2 + I3 + I4 + I5 + c2^2*m2 + c3^2*m3 + c4^2*m4 + c5^2*m5 + l2^2*m2 + l2^2*m3 + l2^2*m4 + l2^2*m5 + l4^2*m5 - 2*c2*l2*m2 + c5*l1*m5*cos(q2 + q3 + q4 + q5) + c3*l1*m3*cos(q2 + q3) + 2*c4*l2*m4*cos(q3 + q4) + 2*l2*l4*m5*cos(q3 + q4) - c2*l1*m2*cos(q2) + 2*c3*l2*m3*cos(q3) + 2*c5*l4*m5*cos(q5) + l1*l2*m2*cos(q2) + l1*l2*m3*cos(q2) + l1*l2*m4*cos(q2) + l1*l2*m5*cos(q2) + c4*l1*m4*cos(q2 + q3 + q4) + 2*c5*l2*m5*cos(q3 + q4 + q5) + l1*l4*m5*cos(q2 + q3 + q4);
    M(1,3) = I3 + I4 + I5 + c3^2*m3 + c4^2*m4 + c5^2*m5 + l4^2*m5 + c5*l1*m5*cos(q2 + q3 + q4 + q5) + c3*l1*m3*cos(q2 + q3) + c4*l2*m4*cos(q3 + q4) + l2*l4*m5*cos(q3 + q4) + c3*l2*m3*cos(q3) + 2*c5*l4*m5*cos(q5) + c4*l1*m4*cos(q2 + q3 + q4) + c5*l2*m5*cos(q3 + q4 + q5) + l1*l4*m5*cos(q2 + q3 + q4);
    M(1,4) = I4 + I5 + c4^2*m4 + c5^2*m5 + l4^2*m5 + c5*l1*m5*cos(q2 + q3 + q4 + q5) + c4*l2*m4*cos(q3 + q4) + l2*l4*m5*cos(q3 + q4) + 2*c5*l4*m5*cos(q5) + c4*l1*m4*cos(q2 + q3 + q4) + c5*l2*m5*cos(q3 + q4 + q5) + l1*l4*m5*cos(q2 + q3 + q4);
    M(1,5) = I5 + c5^2*m5 + c5*l1*m5*cos(q2 + q3 + q4 + q5) + c5*l4*m5*cos(q5) + c5*l2*m5*cos(q3 + q4 + q5);
    M(2,1) = I2 + I3 + I4 + I5 + c2^2*m2 + c3^2*m3 + c4^2*m4 + c5^2*m5 + l2^2*m2 + l2^2*m3 + l2^2*m4 + l2^2*m5 + l4^2*m5 - 2*c2*l2*m2 + c5*l1*m5*cos(q2 + q3 + q4 + q5) + c3*l1*m3*cos(q2 + q3) + 2*c4*l2*m4*cos(q3 + q4) + 2*l2*l4*m5*cos(q3 + q4) - c2*l1*m2*cos(q2) + 2*c3*l2*m3*cos(q3) + 2*c5*l4*m5*cos(q5) + l1*l2*m2*cos(q2) + l1*l2*m3*cos(q2) + l1*l2*m4*cos(q2) + l1*l2*m5*cos(q2) + c4*l1*m4*cos(q2 + q3 + q4) + 2*c5*l2*m5*cos(q3 + q4 + q5) + l1*l4*m5*cos(q2 + q3 + q4);
    M(2,2) = I2 + I3 + I4 + I5 + c2^2*m2 + c3^2*m3 + c4^2*m4 + c5^2*m5 + l2^2*m2 + l2^2*m3 + l2^2*m4 + l2^2*m5 + l4^2*m5 - 2*c2*l2*m2 + 2*c4*l2*m4*cos(q3 + q4) + 2*l2*l4*m5*cos(q3 + q4) + 2*c3*l2*m3*cos(q3) + 2*c5*l4*m5*cos(q5) + 2*c5*l2*m5*cos(q3 + q4 + q5);
    M(2,3) = I3 + I4 + I5 + m3*c3^2 + l2*m3*cos(q3)*c3 + m4*c4^2 + l2*m4*cos(q3 + q4)*c4 + m5*c5^2 + 2*m5*cos(q5)*c5*l4 + l2*m5*cos(q3 + q4 + q5)*c5 + m5*l4^2 + l2*m5*cos(q3 + q4)*l4;
    M(2,4) = I4 + I5 + m4*c4^2 + l2*m4*cos(q3 + q4)*c4 + m5*c5^2 + 2*m5*cos(q5)*c5*l4 + l2*m5*cos(q3 + q4 + q5)*c5 + m5*l4^2 + l2*m5*cos(q3 + q4)*l4;
    M(2,5) = I5 + c5^2*m5 + c5*l4*m5*cos(q5) + c5*l2*m5*cos(q3 + q4 + q5);
    M(3,1) = I3 + I4 + I5 + c3^2*m3 + c4^2*m4 + c5^2*m5 + l4^2*m5 + c5*l1*m5*cos(q2 + q3 + q4 + q5) + c3*l1*m3*cos(q2 + q3) + c4*l2*m4*cos(q3 + q4) + l2*l4*m5*cos(q3 + q4) + c3*l2*m3*cos(q3) + 2*c5*l4*m5*cos(q5) + c4*l1*m4*cos(q2 + q3 + q4) + c5*l2*m5*cos(q3 + q4 + q5) + l1*l4*m5*cos(q2 + q3 + q4);
    M(3,2) = I3 + I4 + I5 + m3*c3^2 + l2*m3*cos(q3)*c3 + m4*c4^2 + l2*m4*cos(q3 + q4)*c4 + m5*c5^2 + 2*m5*cos(q5)*c5*l4 + l2*m5*cos(q3 + q4 + q5)*c5 + m5*l4^2 + l2*m5*cos(q3 + q4)*l4;
    M(3,3) = I3 + I4 + I5 + m3*c3^2 + m4*c4^2 + m5*c5^2 + 2*m5*cos(q5)*c5*l4 + m5*l4^2;
    M(3,4) = I4 + I5 + m4*c4^2 + m5*c5^2 + 2*m5*cos(q5)*c5*l4 + m5*l4^2;
    M(3,5) = I5 + m5*c5^2 + l4*m5*cos(q5)*c5;
    M(4,1) = I4 + I5 + c4^2*m4 + c5^2*m5 + l4^2*m5 + c5*l1*m5*cos(q2 + q3 + q4 + q5) + c4*l2*m4*cos(q3 + q4) + l2*l4*m5*cos(q3 + q4) + 2*c5*l4*m5*cos(q5) + c4*l1*m4*cos(q2 + q3 + q4) + c5*l2*m5*cos(q3 + q4 + q5) + l1*l4*m5*cos(q2 + q3 + q4);
    M(4,2) = I4 + I5 + m4*c4^2 + l2*m4*cos(q3 + q4)*c4 + m5*c5^2 + 2*m5*cos(q5)*c5*l4 + l2*m5*cos(q3 + q4 + q5)*c5 + m5*l4^2 + l2*m5*cos(q3 + q4)*l4;
    M(4,3) = I4 + I5 + m4*c4^2 + m5*c5^2 + 2*m5*cos(q5)*c5*l4 + m5*l4^2;
    M(4,4) = I4 + I5 + m4*c4^2 + m5*c5^2 + 2*m5*cos(q5)*c5*l4 + m5*l4^2;
    M(4,5) = I5 + m5*c5^2 + l4*m5*cos(q5)*c5;
    M(5,1) = I5 + c5^2*m5 + c5*l1*m5*cos(q2 + q3 + q4 + q5) + c5*l4*m5*cos(q5) + c5*l2*m5*cos(q3 + q4 + q5);
    M(5,2) = I5 + c5^2*m5 + c5*l4*m5*cos(q5) + c5*l2*m5*cos(q3 + q4 + q5);
    M(5,3) = I5 + m5*c5^2 + l4*m5*cos(q5)*c5;
    M(5,4) = I5 + m5*c5^2 + l4*m5*cos(q5)*c5;
    M(5,5) = I5 + m5*c5^2;
  
    G(1) = g*(m3*(l2*cos(q1 + q2) + l1*cos(q1) + c3*cos(q1 + q2 + q3)) + m5*(l4*cos(q1 + q2 + q3 + q4) + l2*cos(q1 + q2) + l1*cos(q1) + c5*cos(q1 + q2 + q3 + q4 + q5)) - m2*(cos(q1 + q2)*(c2 - l2) - l1*cos(q1)) + m4*(c4*cos(q1 + q2 + q3 + q4) + l2*cos(q1 + q2) + l1*cos(q1)) - m1*cos(q1)*(c1 - l1));
    G(2) = g*(m3*(l2*cos(q1 + q2) + c3*cos(q1 + q2 + q3)) + m5*(l4*cos(q1 + q2 + q3 + q4) + l2*cos(q1 + q2) + c5*cos(q1 + q2 + q3 + q4 + q5)) + m4*(c4*cos(q1 + q2 + q3 + q4) + l2*cos(q1 + q2)) - m2*cos(q1 + q2)*(c2 - l2));
    G(3) = g*(m5*(l4*cos(q1 + q2 + q3 + q4) + c5*cos(q1 + q2 + q3 + q4 + q5)) + c3*m3*cos(q1 + q2 + q3) + c4*m4*cos(q1 + q2 + q3 + q4));
    G(4) = g*(m5*(l4*cos(q1 + q2 + q3 + q4) + c5*cos(q1 + q2 + q3 + q4 + q5)) + c4*m4*cos(q1 + q2 + q3 + q4));
    G(5) = g*c5*m5*cos(q1 + q2 + q3 + q4 + q5);
    
    C(1) = c2*dq2^2*l1*m2*sin(q2) - c3*dq3^2*l1*m3*sin(q2 + q3) - c4*dq3^2*l2*m4*sin(q3 + q4) - c4*dq4^2*l2*m4*sin(q3 + q4) - dq3^2*l2*l4*m5*sin(q3 + q4) - dq4^2*l2*l4*m5*sin(q3 + q4) - c3*dq2^2*l1*m3*sin(q2 + q3) - c3*dq3^2*l2*m3*sin(q3) - c5*dq5^2*l4*m5*sin(q5) - dq2^2*l1*l2*m2*sin(q2) - dq2^2*l1*l2*m3*sin(q2) - dq2^2*l1*l2*m4*sin(q2) - dq2^2*l1*l2*m5*sin(q2) - c4*dq2^2*l1*m4*sin(q2 + q3 + q4) - c4*dq3^2*l1*m4*sin(q2 + q3 + q4) - c4*dq4^2*l1*m4*sin(q2 + q3 + q4) - c5*dq3^2*l2*m5*sin(q3 + q4 + q5) - c5*dq4^2*l2*m5*sin(q3 + q4 + q5) - c5*dq5^2*l2*m5*sin(q3 + q4 + q5) - dq2^2*l1*l4*m5*sin(q2 + q3 + q4) - dq3^2*l1*l4*m5*sin(q2 + q3 + q4) - dq4^2*l1*l4*m5*sin(q2 + q3 + q4) - c5*dq2^2*l1*m5*sin(q2 + q3 + q4 + q5) - c5*dq3^2*l1*m5*sin(q2 + q3 + q4 + q5) - c5*dq4^2*l1*m5*sin(q2 + q3 + q4 + q5) - c5*dq5^2*l1*m5*sin(q2 + q3 + q4 + q5) - 2*c3*dq1*dq2*l1*m3*sin(q2 + q3) - 2*c3*dq1*dq3*l1*m3*sin(q2 + q3) - 2*c3*dq2*dq3*l1*m3*sin(q2 + q3) - 2*c4*dq1*dq3*l2*m4*sin(q3 + q4) - 2*c4*dq1*dq4*l2*m4*sin(q3 + q4) - 2*c4*dq2*dq3*l2*m4*sin(q3 + q4) - 2*c4*dq2*dq4*l2*m4*sin(q3 + q4) - 2*c4*dq3*dq4*l2*m4*sin(q3 + q4) - 2*dq1*dq3*l2*l4*m5*sin(q3 + q4) - 2*dq1*dq4*l2*l4*m5*sin(q3 + q4) - 2*dq2*dq3*l2*l4*m5*sin(q3 + q4) - 2*dq2*dq4*l2*l4*m5*sin(q3 + q4) - 2*dq3*dq4*l2*l4*m5*sin(q3 + q4) + 2*c2*dq1*dq2*l1*m2*sin(q2) - 2*c3*dq1*dq3*l2*m3*sin(q3) - 2*c3*dq2*dq3*l2*m3*sin(q3) - 2*c5*dq1*dq5*l4*m5*sin(q5) - 2*c5*dq2*dq5*l4*m5*sin(q5) - 2*c5*dq3*dq5*l4*m5*sin(q5) - 2*c5*dq4*dq5*l4*m5*sin(q5) - 2*dq1*dq2*l1*l2*m2*sin(q2) - 2*dq1*dq2*l1*l2*m3*sin(q2) - 2*dq1*dq2*l1*l2*m4*sin(q2) - 2*dq1*dq2*l1*l2*m5*sin(q2) - 2*c4*dq1*dq2*l1*m4*sin(q2 + q3 + q4) - 2*c4*dq1*dq3*l1*m4*sin(q2 + q3 + q4) - 2*c4*dq1*dq4*l1*m4*sin(q2 + q3 + q4) - 2*c4*dq2*dq3*l1*m4*sin(q2 + q3 + q4) - 2*c4*dq2*dq4*l1*m4*sin(q2 + q3 + q4) - 2*c4*dq3*dq4*l1*m4*sin(q2 + q3 + q4) - 2*c5*dq1*dq3*l2*m5*sin(q3 + q4 + q5) - 2*c5*dq1*dq4*l2*m5*sin(q3 + q4 + q5) - 2*c5*dq2*dq3*l2*m5*sin(q3 + q4 + q5) - 2*c5*dq1*dq5*l2*m5*sin(q3 + q4 + q5) - 2*c5*dq2*dq4*l2*m5*sin(q3 + q4 + q5) - 2*c5*dq2*dq5*l2*m5*sin(q3 + q4 + q5) - 2*c5*dq3*dq4*l2*m5*sin(q3 + q4 + q5) - 2*c5*dq3*dq5*l2*m5*sin(q3 + q4 + q5) - 2*c5*dq4*dq5*l2*m5*sin(q3 + q4 + q5) - 2*dq1*dq2*l1*l4*m5*sin(q2 + q3 + q4) - 2*dq1*dq3*l1*l4*m5*sin(q2 + q3 + q4) - 2*dq1*dq4*l1*l4*m5*sin(q2 + q3 + q4) - 2*dq2*dq3*l1*l4*m5*sin(q2 + q3 + q4) - 2*dq2*dq4*l1*l4*m5*sin(q2 + q3 + q4) - 2*dq3*dq4*l1*l4*m5*sin(q2 + q3 + q4) - 2*c5*dq1*dq2*l1*m5*sin(q2 + q3 + q4 + q5) - 2*c5*dq1*dq3*l1*m5*sin(q2 + q3 + q4 + q5) - 2*c5*dq1*dq4*l1*m5*sin(q2 + q3 + q4 + q5) - 2*c5*dq2*dq3*l1*m5*sin(q2 + q3 + q4 + q5) - 2*c5*dq1*dq5*l1*m5*sin(q2 + q3 + q4 + q5) - 2*c5*dq2*dq4*l1*m5*sin(q2 + q3 + q4 + q5) - 2*c5*dq2*dq5*l1*m5*sin(q2 + q3 + q4 + q5) - 2*c5*dq3*dq4*l1*m5*sin(q2 + q3 + q4 + q5) - 2*c5*dq3*dq5*l1*m5*sin(q2 + q3 + q4 + q5) - 2*c5*dq4*dq5*l1*m5*sin(q2 + q3 + q4 + q5);
    C(2) = c3*dq1^2*l1*m3*sin(q2 + q3) - c4*dq3^2*l2*m4*sin(q3 + q4) - c4*dq4^2*l2*m4*sin(q3 + q4) - dq3^2*l2*l4*m5*sin(q3 + q4) - dq4^2*l2*l4*m5*sin(q3 + q4) - c2*dq1^2*l1*m2*sin(q2) - c3*dq3^2*l2*m3*sin(q3) - c5*dq5^2*l4*m5*sin(q5) + dq1^2*l1*l2*m2*sin(q2) + dq1^2*l1*l2*m3*sin(q2) + dq1^2*l1*l2*m4*sin(q2) + dq1^2*l1*l2*m5*sin(q2) + c4*dq1^2*l1*m4*sin(q2 + q3 + q4) - c5*dq3^2*l2*m5*sin(q3 + q4 + q5) - c5*dq4^2*l2*m5*sin(q3 + q4 + q5) - c5*dq5^2*l2*m5*sin(q3 + q4 + q5) + dq1^2*l1*l4*m5*sin(q2 + q3 + q4) + c5*dq1^2*l1*m5*sin(q2 + q3 + q4 + q5) - 2*c4*dq1*dq3*l2*m4*sin(q3 + q4) - 2*c4*dq1*dq4*l2*m4*sin(q3 + q4) - 2*c4*dq2*dq3*l2*m4*sin(q3 + q4) - 2*c4*dq2*dq4*l2*m4*sin(q3 + q4) - 2*c4*dq3*dq4*l2*m4*sin(q3 + q4) - 2*dq1*dq3*l2*l4*m5*sin(q3 + q4) - 2*dq1*dq4*l2*l4*m5*sin(q3 + q4) - 2*dq2*dq3*l2*l4*m5*sin(q3 + q4) - 2*dq2*dq4*l2*l4*m5*sin(q3 + q4) - 2*dq3*dq4*l2*l4*m5*sin(q3 + q4) - 2*c3*dq1*dq3*l2*m3*sin(q3) - 2*c3*dq2*dq3*l2*m3*sin(q3) - 2*c5*dq1*dq5*l4*m5*sin(q5) - 2*c5*dq2*dq5*l4*m5*sin(q5) - 2*c5*dq3*dq5*l4*m5*sin(q5) - 2*c5*dq4*dq5*l4*m5*sin(q5) - 2*c5*dq1*dq3*l2*m5*sin(q3 + q4 + q5) - 2*c5*dq1*dq4*l2*m5*sin(q3 + q4 + q5) - 2*c5*dq2*dq3*l2*m5*sin(q3 + q4 + q5) - 2*c5*dq1*dq5*l2*m5*sin(q3 + q4 + q5) - 2*c5*dq2*dq4*l2*m5*sin(q3 + q4 + q5) - 2*c5*dq2*dq5*l2*m5*sin(q3 + q4 + q5) - 2*c5*dq3*dq4*l2*m5*sin(q3 + q4 + q5) - 2*c5*dq3*dq5*l2*m5*sin(q3 + q4 + q5) - 2*c5*dq4*dq5*l2*m5*sin(q3 + q4 + q5);
    C(3) = c3*dq1^2*l1*m3*sin(q2 + q3) + c4*dq1^2*l2*m4*sin(q3 + q4) + c4*dq2^2*l2*m4*sin(q3 + q4) + dq1^2*l2*l4*m5*sin(q3 + q4) + dq2^2*l2*l4*m5*sin(q3 + q4) + c3*dq1^2*l2*m3*sin(q3) + c3*dq2^2*l2*m3*sin(q3) - c5*dq5^2*l4*m5*sin(q5) + c4*dq1^2*l1*m4*sin(q2 + q3 + q4) + c5*dq1^2*l2*m5*sin(q3 + q4 + q5) + c5*dq2^2*l2*m5*sin(q3 + q4 + q5) + dq1^2*l1*l4*m5*sin(q2 + q3 + q4) + c5*dq1^2*l1*m5*sin(q2 + q3 + q4 + q5) + 2*c4*dq1*dq2*l2*m4*sin(q3 + q4) + 2*dq1*dq2*l2*l4*m5*sin(q3 + q4) + 2*c3*dq1*dq2*l2*m3*sin(q3) - 2*c5*dq1*dq5*l4*m5*sin(q5) - 2*c5*dq2*dq5*l4*m5*sin(q5) - 2*c5*dq3*dq5*l4*m5*sin(q5) - 2*c5*dq4*dq5*l4*m5*sin(q5) + 2*c5*dq1*dq2*l2*m5*sin(q3 + q4 + q5);
    C(4) = c4*dq1^2*l2*m4*sin(q3 + q4) + c4*dq2^2*l2*m4*sin(q3 + q4) + dq1^2*l2*l4*m5*sin(q3 + q4) + dq2^2*l2*l4*m5*sin(q3 + q4) - c5*dq5^2*l4*m5*sin(q5) + c4*dq1^2*l1*m4*sin(q2 + q3 + q4) + c5*dq1^2*l2*m5*sin(q3 + q4 + q5) + c5*dq2^2*l2*m5*sin(q3 + q4 + q5) + dq1^2*l1*l4*m5*sin(q2 + q3 + q4) + c5*dq1^2*l1*m5*sin(q2 + q3 + q4 + q5) + 2*c4*dq1*dq2*l2*m4*sin(q3 + q4) + 2*dq1*dq2*l2*l4*m5*sin(q3 + q4) - 2*c5*dq1*dq5*l4*m5*sin(q5) - 2*c5*dq2*dq5*l4*m5*sin(q5) - 2*c5*dq3*dq5*l4*m5*sin(q5) - 2*c5*dq4*dq5*l4*m5*sin(q5) + 2*c5*dq1*dq2*l2*m5*sin(q3 + q4 + q5);
    C(5) = c5*m5*(dq1^2*l1*sin(q2 + q3 + q4 + q5) + dq1^2*l4*sin(q5) + dq2^2*l4*sin(q5) + dq3^2*l4*sin(q5) + dq4^2*l4*sin(q5) + dq1^2*l2*sin(q3 + q4 + q5) + dq2^2*l2*sin(q3 + q4 + q5) + 2*dq1*dq2*l4*sin(q5) + 2*dq1*dq3*l4*sin(q5) + 2*dq1*dq4*l4*sin(q5) + 2*dq2*dq3*l4*sin(q5) + 2*dq2*dq4*l4*sin(q5) + 2*dq3*dq4*l4*sin(q5) + 2*dq1*dq2*l2*sin(q3 + q4 + q5));
    
    Qext(1) = F11 + F10*l5*cos(q1 + q2 + q3 + q4 + q5) - F9*l5*sin(q1 + q2 + q3 + q4 + q5) + F6*l3*cos(q1 + q2 + q3) - F5*l3*sin(q1 + q2 + q3) + F8*l4*cos(q1 + q2 + q3 + q4) + F10*l4*cos(q1 + q2 + q3 + q4) - F7*l4*sin(q1 + q2 + q3 + q4) - F9*l4*sin(q1 + q2 + q3 + q4) + F4*l2*cos(q1 + q2) + F6*l2*cos(q1 + q2) + F8*l2*cos(q1 + q2) + F10*l2*cos(q1 + q2) - F3*l2*sin(q1 + q2) - F5*l2*sin(q1 + q2) - F7*l2*sin(q1 + q2) - F9*l2*sin(q1 + q2) + F2*l1*cos(q1) + F4*l1*cos(q1) + F6*l1*cos(q1) + F8*l1*cos(q1) + F10*l1*cos(q1) - F1*l1*sin(q1) - F3*l1*sin(q1) - F5*l1*sin(q1) - F7*l1*sin(q1) - F9*l1*sin(q1);
    Qext(2) = F12 + F10*l5*cos(q1 + q2 + q3 + q4 + q5) - F9*l5*sin(q1 + q2 + q3 + q4 + q5) + F6*l3*cos(q1 + q2 + q3) - F5*l3*sin(q1 + q2 + q3) + F8*l4*cos(q1 + q2 + q3 + q4) + F10*l4*cos(q1 + q2 + q3 + q4) - F7*l4*sin(q1 + q2 + q3 + q4) - F9*l4*sin(q1 + q2 + q3 + q4) + F4*l2*cos(q1 + q2) + F6*l2*cos(q1 + q2) + F8*l2*cos(q1 + q2) + F10*l2*cos(q1 + q2) - F3*l2*sin(q1 + q2) - F5*l2*sin(q1 + q2) - F7*l2*sin(q1 + q2) - F9*l2*sin(q1 + q2);
    Qext(3) = F13 + F10*(l4*cos(q1 + q2 + q3 + q4) + l5*cos(q1 + q2 + q3 + q4 + q5)) - F9*(l4*sin(q1 + q2 + q3 + q4) + l5*sin(q1 + q2 + q3 + q4 + q5)) + F6*l3*cos(q1 + q2 + q3) - F5*l3*sin(q1 + q2 + q3) + F8*l4*cos(q1 + q2 + q3 + q4) - F7*l4*sin(q1 + q2 + q3 + q4);
    Qext(4) = F14 + F10*(l4*cos(q1 + q2 + q3 + q4) + l5*cos(q1 + q2 + q3 + q4 + q5)) - F9*(l4*sin(q1 + q2 + q3 + q4) + l5*sin(q1 + q2 + q3 + q4 + q5)) + F8*l4*cos(q1 + q2 + q3 + q4) - F7*l4*sin(q1 + q2 + q3 + q4);
    Qext(5) = F15 + F10*l5*cos(q1 + q2 + q3 + q4 + q5) - F9*l5*sin(q1 + q2 + q3 + q4 + q5);
    
    
    %%% Torque Atuante nas Juntas
    %The first component of the Torque is always zero. For simplicity sake,
    %to use the same code we already have, it is already set to be zero on
    %the controller.
    
    Ut = U - [0;dq2;dq3;dq4;dq5]*Cphi;
    
    Fclean = Ut - C - G;
    F = Fclean + Qext;
    
    ddQ = M\F;
    
    momentum = M*[dq1; dq2; dq3; dq4; dq5];
end

== matlab function FeedbackLin/Fext ==
  data: Fext output; dQ input; Q input; t input; pertStep parameter; pertAmp parameter; pertDur parameter; curStep parameter
function Fext = calcFext(dQ, Q, t, pertStep, pertAmp, pertDur, curStep)
    % Adds a constant push at the hip at the beginnning of the desired step.
    % The Fx at the hip is the Fext(3)
    
    Fext = zeros(15,1);
    if(ismember(curStep, pertStep)) %Checks if we want a push at the current step
        if(t <= pertDur)            %Checks if we are still in the duration of the desired push
            Fext(3) = pertAmp;      %Applies an heaviside-like push of amp pertAmp at the hip
        end
    end
end

== matlab function FeedbackLin/Calc Y & xCoM ==
  data: Q input; Y output; xCoM output; cm parameter; mm parameter; lm parameter
function [Y, xCoM] = getOutput(Q, cm, mm, lm)
    %Parameters
    c1 = cm(1);
    c2 = cm(2);
    c3 = cm(3);
    c4 = cm(4);
    c5 = cm(5);
    
    l1 = lm(1);
    l2 = lm(2);
    l3 = lm(3);
    l4 = lm(4);
    l5 = lm(5);
    
    m1 = mm(1);
    m2 = mm(2);
    m3 = mm(3);
    m4 = mm(4);
    m5 = mm(5);
    
    %Position and velocities
    q1 = Q(1);
    q2 = Q(2);
    q3 = Q(3);
    q4 = Q(4);
    q5 = Q(5);
    
    %Auxiliary positions
    O = [0, 0];
    
    A  = O + l1*[cos(q1), sin(q1)];
    B  = A + l2*[cos(q1+q2), sin(q1+q2)];
    C  = B + l4*[cos(q1+q2+q3+q4), sin(q1+q2+q3+q4)];

    P1 = O + (l1-c1)*[cos(q1), sin(q1)];
    P2 = A + (l2-c2)*[cos(q1+q2), sin(q1+q2)];
    P3 = B + c3*[cos(q1+q2+q3), sin(q1+q2+q3)];
    P4 = B + c4*[cos(q1+q2+q3+q4), sin(q1+q2+q3+q4)];
    P5 = C + c5*[cos(q1+q2+q3+q4+q5), sin(q1+q2+q3+q4+q5)];
    
    %Computes outputs
    CoM = (m1*P1 + m2*P2 + m3*P3 + m4*P4 + m5*P5)/(m1+m2+m3+m4+m5); 
    PSW = C + l5*[cos(q1+q2+q3+q4+q5), sin(q1+q2+q3+q4+q5)];
    QT = (5*pi/2) - q1 - q2 - q3;
    
    %Constructs the output
    Y = [QT;
         PSW(2);
         CoM(2);
         PSW(1)];
     
    xCoM = CoM(1);
end

== matlab function FeedbackLin/calch0 ==
  data: Q input; h0 output; lr parameter; mInc parameter
function h0 = calch0(Q, lr, mInc)

    q1 = Q(1);
    q2 = Q(2);
    q3 = Q(3);
    q4 = Q(4);
    q5 = Q(5);

    l1 = lr(1);
    l2 = lr(2);
    l3 = lr(3);
    l4 = lr(4);
    l5 = lr(5);
    
    
    SWx = l1*cos(q1) + l2*cos(q1 + q2) + l4*cos(q1 + q2 + q3 + q4) + l5*cos(q1 + q2 + q3 + q4 + q5);
    h0 = mInc*SWx;
end

== matlab function FeedbackLin/Detec Impact/Impact ==
  data: dQ input; dQp output; Q input; Qp output; h0 input; lr parameter; Imp output; t input; SWy output
function [dQp, Qp, Imp, SWy] = checkImpact(dQ, Q, h0, lr, t)

    margin = 0;

    l1 = lr(1);
    l2 = lr(2);
    l3 = lr(3);
    l4 = lr(4);
    l5 = lr(5);
    
    q1 = Q(1);
    q2 = Q(2);
    q3 = Q(3);
    q4 = Q(4);
    q5 = Q(5);
        
    SWy = l1*sin(q1) + l2*sin(q1 + q2) + l4*sin(q1 + q2 + q3 + q4) + l5*sin(q1 + q2 + q3 + q4 + q5);
    
    Qp  = Q;
    dQp = dQ;
    
    if(SWy <= (h0+margin) && (t>0.05))
        Imp = 1;
    else
        Imp = 0;
    end
end

== matlab function FeedbackLin/getDesiredCoords/High Level Controller - Cycloidal1 ==
  data: dQ input; Q input; Yd output; t input; dYd output; ddYd output; Tpasso parameter
function [Yd, dYd, ddYd] = HighLevel(dQ, Q, t, Tpasso)
    %Rstep should be calculated from the capture point. Rember here that
    %the total length of the step is divided half before the stance feet
    %(origin of the system) and half after the stance feet. So the Rstep
    %should be twice the desired step position that comes from the capture
    %point. We will calculate de prediction of the capture point at the end
    %of the step and gradually update our Rstep to its value.
    Tref   = Tpasso;    %Seconds. Ref =  Hip
    Taux   = Tpasso;    %Seconds. Aux = Trunk oscillation

    Aaux   = 0;         %The trunk inclination is defined as a constant plus a
    phiaux = 0;         %sine according to the following equation:
    aux0 = 10*pi/180;   %aux0 + Aaux*sin(waux*T + phiaux), in rads.
    Yrefh  = 0.7;       %Height to be maintained by the hip.
    Rstep  = 0.7;       %Length of a step in m.
    
    w = 2*pi/Tpasso;
    Vref = Rstep/(2*Tref);
    waux = 2*pi/Taux;

    Rref = Rstep/4;
    r = Rstep/(2*pi);
    
    THETA = w*t;
    
    if(t < 10*Tpasso)
        xsw = -(Rstep/2) + r*(THETA - sin(THETA));
        ysw = r*(1 - cos(THETA));
        xh = -Rref + Vref*t;
        yh = Yrefh;
        qt = aux0 + Aaux*sin(waux*t + phiaux);

        dxsw = r*w*(1 - cos(THETA));
        dysw = r*w*(sin(THETA));
        dxh = Vref;
        dyh = 0;
        dqt = Aaux*waux*cos(waux*t + phiaux);

        ddxsw = r*w^2*(sin(THETA));
        ddysw = r*w^2*(cos(THETA));
        ddxh = 0;
        ddyh = 0;
        ddqt = -Aaux*waux^2*sin(waux*t + phiaux);
    else
        xsw = Rstep/2;
        ysw = ((-r*w^2)/2)*(t-Tpasso)^2;
        xh = Rref;
        yh = Yrefh;
        qt = aux0 + Aaux*sin(waux*t + phiaux);

        dxsw = 0;
        dysw = (-r*w^2)*(t-Tpasso);
        dxh  = 0;
        dyh  = 0;
        dqt  = 0;

        ddxsw = 0;
        ddysw = -r*w^2;
        ddxh  = 0;
        ddyh  = 0;
        ddqt  = 0;
    end
%     XSW = [xsw; dxsw; ddxsw];
%     YSW = [ysw; dysw; ddysw];
%     XH  = [xh; dxh; ddxh];
%     YH  = [yh; dyh; ddyh];
%     QT  = [qt; dqt; ddqt];
    
    Yd   = [  qt;   ysw;   yh;   xsw];
    dYd  = [ dqt;  dysw;  dyh;  dxsw];
    ddYd = [ddqt; ddysw; ddyh; ddxsw];
end
